simulink model "sistema_only_master"  (R2015a)
settings: Solver=ode45  StartTime=0.0  StopTime=10  RelTol=1e-3
values from neighbouring files (symbols this model uses):
  A_master = [0 1; 0 -Bm/Mm]    [init_model.m]    (also in init_model_only_master.m)
  B_master = [0; 1/Mm]    [init_model.m]    (also in init_model_only_master.m)
  C_master = [1 0; 0 1]    [init_model.m]    (also in init_model_only_master.m)
  D_master = [0; 0]    [init_model.m]    (also in init_model_only_master.m)
  K = [ ... (first row only)    [init_model.m]    (also in init_model_only_master.m = [-19.9294    1.9743]; robustlqr.m = value(L)*inv(value(Y)))
settings Model: Creator=enrico-giordano  LastModifiedBy=enrico-giordano

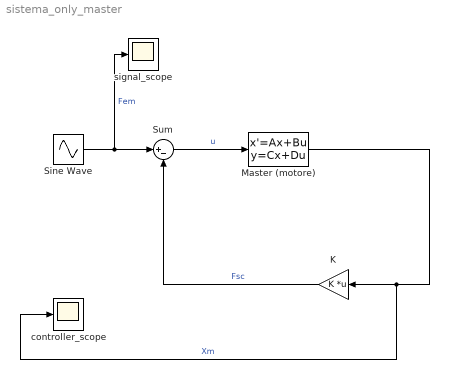
== system sistema_only_master ==
  K : Gain  Gain=K  Multiplication=Matrix(K*u)
  Master (motore) : StateSpace  A=A_master  B=B_master  C=C_master  D=D_master  X0=0
  Sine Wave : Sin  Amplitude=10  SampleTime=0
  Sum : Sum  Inputs=|+-
  controller_scope : Scope
      settings: TimeRange=10  YMin=-0.6000000000000001  YMax=0.2  SaveName=ScopeData3
  signal_scope : Scope
      settings: TimeRange=10  YMin=-10  YMax=10
  wires:
  Sum/1 -> Master (motore)/1  "u"
  Sine Wave/1 -> signal_scope/1, Sum/1  "Fem"
  Master (motore)/1 -> controller_scope/1, K/1  "Xm"
  K/1 -> Sum/2  "Fsc"
